simulink model "section_6_2_second_group"  (R2020a)
settings: Solver=ode45  StartTime=0.0  StopTime=50  RelTol=1e-5  EnableMultiTasking=on
(part 2 of 4)

== matlab function section_6_2_second_group/FUZZY3/fuzzy_logic_system1 ==
  data: aF output; x1 input; x2 input; x3 input; w input
function aF    = fcn(x1,x2,x3,w)
%%x1 5条模糊规则
delta=0.01;
ux1=zeros(5,1);
ux2=zeros(5,1);
ux3=zeros(5,1);
%%x1 5条模糊规则

h1=1;%%规则间距
if x1<=-2-delta
    ux1(1,1)=1;
end

if x1>=-2-delta&&x1<=-1-delta
    ux1(1,1)=0.5*sin(pi*(x1-(-2-delta))/h1+0.5*pi)+0.5;
end

if x1>=-2-delta&&x1<=0-delta
    ux1(2,1)=0.5*sin(pi*(x1-(-1-delta))/h1+0.5*pi)+0.5;
end

if x1>=-1-delta&&x1<=1-delta
    ux1(3,1)=0.5*sin(pi*(x1-(0-delta))/h1+0.5*pi)+0.5;
end

if x1>=0-delta&&x1<=2-delta
    ux1(4,1)=0.5*sin(pi*(x1-(1-delta))/h1+0.5*pi)+0.5;
end

if x1>=1-delta&&x1<=2-delta
    ux1(5,1)=0.5*sin(pi*(x1-(2-delta))/h1+0.5*pi)+0.5;
end

if x1>2-delta
    ux1(5,1)=1;
end


h2=1;%%规则间距
if x2<=-2-delta
    ux2(1,1)=1;
end

if x2>=-2-delta&&x2<=-1-delta
    ux2(1,1)=0.5*sin(pi*(x2-(-2-delta))/h2+0.5*pi)+0.5;
end

if x2>=-2-delta&&x2<=0-delta
    ux2(2,1)=0.5*sin(pi*(x2-(-1-delta))/h2+0.5*pi)+0.5;
end

if x2>=-1-delta&&x2<=1-delta
    ux2(3,1)=0.5*sin(pi*(x2-(0-delta))/h2+0.5*pi)+0.5;
end

if x2>=0-delta&&x2<=2-delta
    ux2(4,1)=0.5*sin(pi*(x2-(1-delta))/h2+0.5*pi)+0.5;
end

if x2>=1-delta&&x2<=2-delta
    ux2(5,1)=0.5*sin(pi*(x2-(2-delta))/h2+0.5*pi)+0.5;
end

if x2>2-delta
    ux2(5,1)=1;
end

h3=1;%%规则间距
if x3<=-2-delta
    ux3(1,1)=1;
end

if x3>=-2-delta&&x3<=-1-delta
    ux3(1,1)=0.5*sin(pi*(x3-(-2-delta))/h3+0.5*pi)+0.5;
end

if x3>=-2-delta&&x3<=0-delta
    ux3(2,1)=0.5*sin(pi*(x3-(-1-delta))/h3+0.5*pi)+0.5;
end

if x3>=-1-delta&&x3<=1-delta
    ux3(3,1)=0.5*sin(pi*(x3-(0-delta))/h3+0.5*pi)+0.5;
end

if x3>=0-delta&&x3<=2-delta
    ux3(4,1)=0.5*sin(pi*(x3-(1-delta))/h3+0.5*pi)+0.5;
end

if x3>=1-delta&&x3<=2-delta
    ux3(5,1)=0.5*sin(pi*(x3-(2-delta))/h3+0.5*pi)+0.5;
end

if x3>2-delta
    ux3(5,1)=1;
end



%中心平均解模糊
Basic=0;
for i1=1:5
    for i2=1:5
        for i3=1:5
            Basic=Basic+ux1(i1,1)*ux2(i2,1)*ux3(i3,1);
        end
    end
end

beta=zeros(5,5,5);
for i1=1:5
    for i2=1:5
        for i3=1:5
            beta(i1,i2,i3)=ux1(i1,1)*ux2(i2,1)*ux3(i3,1)/Basic;
        end
    end
end


aF=0;
for i1=1:5
    for i2=1:5
        for i3=1:5
            aF=aF+w(i1,i2,i3)*beta(i1,i2,i3); 
        end
    end
end

end

== matlab function section_6_2_second_group/FUZZY3/fuzzy_logic_system10 ==
  data: aF output; x1 input; x2 input; x3 input; w input
function aF    = fcn(x1,x2,x3,w)
%%x1 5条模糊规则
delta=0.01;
ux1=zeros(5,1);
ux2=zeros(5,1);
ux3=zeros(5,1);
%%x1 5条模糊规则

h1=1;%%规则间距
if x1<=-2-delta
    ux1(1,1)=1;
end

if x1>=-2-delta&&x1<=-1-delta
    ux1(1,1)=0.5*sin(pi*(x1-(-2-delta))/h1+0.5*pi)+0.5;
end

if x1>=-2-delta&&x1<=0-delta
    ux1(2,1)=0.5*sin(pi*(x1-(-1-delta))/h1+0.5*pi)+0.5;
end

if x1>=-1-delta&&x1<=1-delta
    ux1(3,1)=0.5*sin(pi*(x1-(0-delta))/h1+0.5*pi)+0.5;
end

if x1>=0-delta&&x1<=2-delta
    ux1(4,1)=0.5*sin(pi*(x1-(1-delta))/h1+0.5*pi)+0.5;
end

if x1>=1-delta&&x1<=2-delta
    ux1(5,1)=0.5*sin(pi*(x1-(2-delta))/h1+0.5*pi)+0.5;
end

if x1>2-delta
    ux1(5,1)=1;
end


h2=1;%%规则间距
if x2<=-2-delta
    ux2(1,1)=1;
end

if x2>=-2-delta&&x2<=-1-delta
    ux2(1,1)=0.5*sin(pi*(x2-(-2-delta))/h2+0.5*pi)+0.5;
end

if x2>=-2-delta&&x2<=0-delta
    ux2(2,1)=0.5*sin(pi*(x2-(-1-delta))/h2+0.5*pi)+0.5;
end

if x2>=-1-delta&&x2<=1-delta
    ux2(3,1)=0.5*sin(pi*(x2-(0-delta))/h2+0.5*pi)+0.5;
end

if x2>=0-delta&&x2<=2-delta
    ux2(4,1)=0.5*sin(pi*(x2-(1-delta))/h2+0.5*pi)+0.5;
end

if x2>=1-delta&&x2<=2-delta
    ux2(5,1)=0.5*sin(pi*(x2-(2-delta))/h2+0.5*pi)+0.5;
end

if x2>2-delta
    ux2(5,1)=1;
end

h3=1;%%规则间距
if x3<=-2-delta
    ux3(1,1)=1;
end

if x3>=-2-delta&&x3<=-1-delta
    ux3(1,1)=0.5*sin(pi*(x3-(-2-delta))/h3+0.5*pi)+0.5;
end

if x3>=-2-delta&&x3<=0-delta
    ux3(2,1)=0.5*sin(pi*(x3-(-1-delta))/h3+0.5*pi)+0.5;
end

if x3>=-1-delta&&x3<=1-delta
    ux3(3,1)=0.5*sin(pi*(x3-(0-delta))/h3+0.5*pi)+0.5;
end

if x3>=0-delta&&x3<=2-delta
    ux3(4,1)=0.5*sin(pi*(x3-(1-delta))/h3+0.5*pi)+0.5;
end

if x3>=1-delta&&x3<=2-delta
    ux3(5,1)=0.5*sin(pi*(x3-(2-delta))/h3+0.5*pi)+0.5;
end

if x3>2-delta
    ux3(5,1)=1;
end



%中心平均解模糊
Basic=0;
for i1=1:5
    for i2=1:5
        for i3=1:5
            Basic=Basic+ux1(i1,1)*ux2(i2,1)*ux3(i3,1);
        end
    end
end

beta=zeros(5,5,5);
for i1=1:5
    for i2=1:5
        for i3=1:5
            beta(i1,i2,i3)=ux1(i1,1)*ux2(i2,1)*ux3(i3,1)/Basic;
        end
    end
end


aF=0;
for i1=1:5
    for i2=1:5
        for i3=1:5
            aF=aF+w(i1,i2,i3)*beta(i1,i2,i3); 
        end
    end
end

end

== matlab function section_6_2_second_group/FUZZY3/fuzzy_logic_system2 ==
  data: aF output; x1 input; x2 input; x3 input; w input
function aF    = fcn(x1,x2,x3,w)
%%x1 5条模糊规则
delta=0.01;
ux1=zeros(5,1);
ux2=zeros(5,1);
ux3=zeros(5,1);
%%x1 5条模糊规则

h1=1;%%规则间距
if x1<=-2-delta
    ux1(1,1)=1;
end

if x1>=-2-delta&&x1<=-1-delta
    ux1(1,1)=0.5*sin(pi*(x1-(-2-delta))/h1+0.5*pi)+0.5;
end

if x1>=-2-delta&&x1<=0-delta
    ux1(2,1)=0.5*sin(pi*(x1-(-1-delta))/h1+0.5*pi)+0.5;
end

if x1>=-1-delta&&x1<=1-delta
    ux1(3,1)=0.5*sin(pi*(x1-(0-delta))/h1+0.5*pi)+0.5;
end

if x1>=0-delta&&x1<=2-delta
    ux1(4,1)=0.5*sin(pi*(x1-(1-delta))/h1+0.5*pi)+0.5;
end

if x1>=1-delta&&x1<=2-delta
    ux1(5,1)=0.5*sin(pi*(x1-(2-delta))/h1+0.5*pi)+0.5;
end

if x1>2-delta
    ux1(5,1)=1;
end


h2=1;%%规则间距
if x2<=-2-delta
    ux2(1,1)=1;
end

if x2>=-2-delta&&x2<=-1-delta
    ux2(1,1)=0.5*sin(pi*(x2-(-2-delta))/h2+0.5*pi)+0.5;
end

if x2>=-2-delta&&x2<=0-delta
    ux2(2,1)=0.5*sin(pi*(x2-(-1-delta))/h2+0.5*pi)+0.5;
end

if x2>=-1-delta&&x2<=1-delta
    ux2(3,1)=0.5*sin(pi*(x2-(0-delta))/h2+0.5*pi)+0.5;
end

if x2>=0-delta&&x2<=2-delta
    ux2(4,1)=0.5*sin(pi*(x2-(1-delta))/h2+0.5*pi)+0.5;
end

if x2>=1-delta&&x2<=2-delta
    ux2(5,1)=0.5*sin(pi*(x2-(2-delta))/h2+0.5*pi)+0.5;
end

if x2>2-delta
    ux2(5,1)=1;
end

h3=1;%%规则间距
if x3<=-2-delta
    ux3(1,1)=1;
end

if x3>=-2-delta&&x3<=-1-delta
    ux3(1,1)=0.5*sin(pi*(x3-(-2-delta))/h3+0.5*pi)+0.5;
end

if x3>=-2-delta&&x3<=0-delta
    ux3(2,1)=0.5*sin(pi*(x3-(-1-delta))/h3+0.5*pi)+0.5;
end

if x3>=-1-delta&&x3<=1-delta
    ux3(3,1)=0.5*sin(pi*(x3-(0-delta))/h3+0.5*pi)+0.5;
end

if x3>=0-delta&&x3<=2-delta
    ux3(4,1)=0.5*sin(pi*(x3-(1-delta))/h3+0.5*pi)+0.5;
end

if x3>=1-delta&&x3<=2-delta
    ux3(5,1)=0.5*sin(pi*(x3-(2-delta))/h3+0.5*pi)+0.5;
end

if x3>2-delta
    ux3(5,1)=1;
end



%中心平均解模糊
Basic=0;
for i1=1:5
    for i2=1:5
        for i3=1:5
            Basic=Basic+ux1(i1,1)*ux2(i2,1)*ux3(i3,1);
        end
    end
end

beta=zeros(5,5,5);
for i1=1:5
    for i2=1:5
        for i3=1:5
            beta(i1,i2,i3)=ux1(i1,1)*ux2(i2,1)*ux3(i3,1)/Basic;
        end
    end
end


aF=0;
for i1=1:5
    for i2=1:5
        for i3=1:5
            aF=aF+w(i1,i2,i3)*beta(i1,i2,i3); 
        end
    end
end

end

== matlab function section_6_2_second_group/FUZZY3/fuzzy_logic_system3 ==
  data: aF output; x1 input; x2 input; x3 input; w input
function aF    = fcn(x1,x2,x3,w)
%%x1 5条模糊规则
delta=0.01;
ux1=zeros(5,1);
ux2=zeros(5,1);
ux3=zeros(5,1);
%%x1 5条模糊规则

h1=1;%%规则间距
if x1<=-2-delta
    ux1(1,1)=1;
end

if x1>=-2-delta&&x1<=-1-delta
    ux1(1,1)=0.5*sin(pi*(x1-(-2-delta))/h1+0.5*pi)+0.5;
end

if x1>=-2-delta&&x1<=0-delta
    ux1(2,1)=0.5*sin(pi*(x1-(-1-delta))/h1+0.5*pi)+0.5;
end

if x1>=-1-delta&&x1<=1-delta
    ux1(3,1)=0.5*sin(pi*(x1-(0-delta))/h1+0.5*pi)+0.5;
end

if x1>=0-delta&&x1<=2-delta
    ux1(4,1)=0.5*sin(pi*(x1-(1-delta))/h1+0.5*pi)+0.5;
end

if x1>=1-delta&&x1<=2-delta
    ux1(5,1)=0.5*sin(pi*(x1-(2-delta))/h1+0.5*pi)+0.5;
end

if x1>2-delta
    ux1(5,1)=1;
end


h2=1;%%规则间距
if x2<=-2-delta
    ux2(1,1)=1;
end

if x2>=-2-delta&&x2<=-1-delta
    ux2(1,1)=0.5*sin(pi*(x2-(-2-delta))/h2+0.5*pi)+0.5;
end

if x2>=-2-delta&&x2<=0-delta
    ux2(2,1)=0.5*sin(pi*(x2-(-1-delta))/h2+0.5*pi)+0.5;
end

if x2>=-1-delta&&x2<=1-delta
    ux2(3,1)=0.5*sin(pi*(x2-(0-delta))/h2+0.5*pi)+0.5;
end

if x2>=0-delta&&x2<=2-delta
    ux2(4,1)=0.5*sin(pi*(x2-(1-delta))/h2+0.5*pi)+0.5;
end

if x2>=1-delta&&x2<=2-delta
    ux2(5,1)=0.5*sin(pi*(x2-(2-delta))/h2+0.5*pi)+0.5;
end

if x2>2-delta
    ux2(5,1)=1;
end

h3=1;%%规则间距
if x3<=-2-delta
    ux3(1,1)=1;
end

if x3>=-2-delta&&x3<=-1-delta
    ux3(1,1)=0.5*sin(pi*(x3-(-2-delta))/h3+0.5*pi)+0.5;
end

if x3>=-2-delta&&x3<=0-delta
    ux3(2,1)=0.5*sin(pi*(x3-(-1-delta))/h3+0.5*pi)+0.5;
end

if x3>=-1-delta&&x3<=1-delta
    ux3(3,1)=0.5*sin(pi*(x3-(0-delta))/h3+0.5*pi)+0.5;
end

if x3>=0-delta&&x3<=2-delta
    ux3(4,1)=0.5*sin(pi*(x3-(1-delta))/h3+0.5*pi)+0.5;
end

if x3>=1-delta&&x3<=2-delta
    ux3(5,1)=0.5*sin(pi*(x3-(2-delta))/h3+0.5*pi)+0.5;
end

if x3>2-delta
    ux3(5,1)=1;
end



%中心平均解模糊
Basic=0;
for i1=1:5
    for i2=1:5
        for i3=1:5
            Basic=Basic+ux1(i1,1)*ux2(i2,1)*ux3(i3,1);
        end
    end
end

beta=zeros(5,5,5);
for i1=1:5
    for i2=1:5
        for i3=1:5
            beta(i1,i2,i3)=ux1(i1,1)*ux2(i2,1)*ux3(i3,1)/Basic;
        end
    end
end


aF=0;
for i1=1:5
    for i2=1:5
        for i3=1:5
            aF=aF+w(i1,i2,i3)*beta(i1,i2,i3); 
        end
    end
end

end

== matlab function section_6_2_second_group/FUZZY3/fuzzy_logic_system4 ==
  data: aF output; x1 input; x2 input; x3 input; w input
function aF    = fcn(x1,x2,x3,w)
%%x1 5条模糊规则
delta=0.01;
ux1=zeros(5,1);
ux2=zeros(5,1);
ux3=zeros(5,1);
%%x1 5条模糊规则

h1=1;%%规则间距
if x1<=-2-delta
    ux1(1,1)=1;
end

if x1>=-2-delta&&x1<=-1-delta
    ux1(1,1)=0.5*sin(pi*(x1-(-2-delta))/h1+0.5*pi)+0.5;
end

if x1>=-2-delta&&x1<=0-delta
    ux1(2,1)=0.5*sin(pi*(x1-(-1-delta))/h1+0.5*pi)+0.5;
end

if x1>=-1-delta&&x1<=1-delta
    ux1(3,1)=0.5*sin(pi*(x1-(0-delta))/h1+0.5*pi)+0.5;
end

if x1>=0-delta&&x1<=2-delta
    ux1(4,1)=0.5*sin(pi*(x1-(1-delta))/h1+0.5*pi)+0.5;
end

if x1>=1-delta&&x1<=2-delta
    ux1(5,1)=0.5*sin(pi*(x1-(2-delta))/h1+0.5*pi)+0.5;
end

if x1>2-delta
    ux1(5,1)=1;
end


h2=1;%%规则间距
if x2<=-2-delta
    ux2(1,1)=1;
end

if x2>=-2-delta&&x2<=-1-delta
    ux2(1,1)=0.5*sin(pi*(x2-(-2-delta))/h2+0.5*pi)+0.5;
end

if x2>=-2-delta&&x2<=0-delta
    ux2(2,1)=0.5*sin(pi*(x2-(-1-delta))/h2+0.5*pi)+0.5;
end

if x2>=-1-delta&&x2<=1-delta
    ux2(3,1)=0.5*sin(pi*(x2-(0-delta))/h2+0.5*pi)+0.5;
end

if x2>=0-delta&&x2<=2-delta
    ux2(4,1)=0.5*sin(pi*(x2-(1-delta))/h2+0.5*pi)+0.5;
end

if x2>=1-delta&&x2<=2-delta
    ux2(5,1)=0.5*sin(pi*(x2-(2-delta))/h2+0.5*pi)+0.5;
end

if x2>2-delta
    ux2(5,1)=1;
end

h3=1;%%规则间距
if x3<=-2-delta
    ux3(1,1)=1;
end

if x3>=-2-delta&&x3<=-1-delta
    ux3(1,1)=0.5*sin(pi*(x3-(-2-delta))/h3+0.5*pi)+0.5;
end

if x3>=-2-delta&&x3<=0-delta
    ux3(2,1)=0.5*sin(pi*(x3-(-1-delta))/h3+0.5*pi)+0.5;
end

if x3>=-1-delta&&x3<=1-delta
    ux3(3,1)=0.5*sin(pi*(x3-(0-delta))/h3+0.5*pi)+0.5;
end

if x3>=0-delta&&x3<=2-delta
    ux3(4,1)=0.5*sin(pi*(x3-(1-delta))/h3+0.5*pi)+0.5;
end

if x3>=1-delta&&x3<=2-delta
    ux3(5,1)=0.5*sin(pi*(x3-(2-delta))/h3+0.5*pi)+0.5;
end

if x3>2-delta
    ux3(5,1)=1;
end



%中心平均解模糊
Basic=0;
for i1=1:5
    for i2=1:5
        for i3=1:5
            Basic=Basic+ux1(i1,1)*ux2(i2,1)*ux3(i3,1);
        end
    end
end

beta=zeros(5,5,5);
for i1=1:5
    for i2=1:5
        for i3=1:5
            beta(i1,i2,i3)=ux1(i1,1)*ux2(i2,1)*ux3(i3,1)/Basic;
        end
    end
end


aF=0;
for i1=1:5
    for i2=1:5
        for i3=1:5
            aF=aF+w(i1,i2,i3)*beta(i1,i2,i3); 
        end
    end
end

end

== matlab function section_6_2_second_group/FUZZY3/fuzzy_logic_system5 ==
  data: aF output; x1 input; x2 input; x3 input; w input
function aF    = fcn(x1,x2,x3,w)
%%x1 5条模糊规则
delta=0.01;
ux1=zeros(5,1);
ux2=zeros(5,1);
ux3=zeros(5,1);
%%x1 5条模糊规则

h1=1;%%规则间距
if x1<=-2-delta
    ux1(1,1)=1;
end

if x1>=-2-delta&&x1<=-1-delta
    ux1(1,1)=0.5*sin(pi*(x1-(-2-delta))/h1+0.5*pi)+0.5;
end

if x1>=-2-delta&&x1<=0-delta
    ux1(2,1)=0.5*sin(pi*(x1-(-1-delta))/h1+0.5*pi)+0.5;
end

if x1>=-1-delta&&x1<=1-delta
    ux1(3,1)=0.5*sin(pi*(x1-(0-delta))/h1+0.5*pi)+0.5;
end

if x1>=0-delta&&x1<=2-delta
    ux1(4,1)=0.5*sin(pi*(x1-(1-delta))/h1+0.5*pi)+0.5;
end

if x1>=1-delta&&x1<=2-delta
    ux1(5,1)=0.5*sin(pi*(x1-(2-delta))/h1+0.5*pi)+0.5;
end

if x1>2-delta
    ux1(5,1)=1;
end


h2=1;%%规则间距
if x2<=-2-delta
    ux2(1,1)=1;
end

if x2>=-2-delta&&x2<=-1-delta
    ux2(1,1)=0.5*sin(pi*(x2-(-2-delta))/h2+0.5*pi)+0.5;
end

if x2>=-2-delta&&x2<=0-delta
    ux2(2,1)=0.5*sin(pi*(x2-(-1-delta))/h2+0.5*pi)+0.5;
end

if x2>=-1-delta&&x2<=1-delta
    ux2(3,1)=0.5*sin(pi*(x2-(0-delta))/h2+0.5*pi)+0.5;
end

if x2>=0-delta&&x2<=2-delta
    ux2(4,1)=0.5*sin(pi*(x2-(1-delta))/h2+0.5*pi)+0.5;
end

if x2>=1-delta&&x2<=2-delta
    ux2(5,1)=0.5*sin(pi*(x2-(2-delta))/h2+0.5*pi)+0.5;
end

if x2>2-delta
    ux2(5,1)=1;
end

h3=1;%%规则间距
if x3<=-2-delta
    ux3(1,1)=1;
end

if x3>=-2-delta&&x3<=-1-delta
    ux3(1,1)=0.5*sin(pi*(x3-(-2-delta))/h3+0.5*pi)+0.5;
end

if x3>=-2-delta&&x3<=0-delta
    ux3(2,1)=0.5*sin(pi*(x3-(-1-delta))/h3+0.5*pi)+0.5;
end

if x3>=-1-delta&&x3<=1-delta
    ux3(3,1)=0.5*sin(pi*(x3-(0-delta))/h3+0.5*pi)+0.5;
end

if x3>=0-delta&&x3<=2-delta
    ux3(4,1)=0.5*sin(pi*(x3-(1-delta))/h3+0.5*pi)+0.5;
end

if x3>=1-delta&&x3<=2-delta
    ux3(5,1)=0.5*sin(pi*(x3-(2-delta))/h3+0.5*pi)+0.5;
end

if x3>2-delta
    ux3(5,1)=1;
end



%中心平均解模糊
Basic=0;
for i1=1:5
    for i2=1:5
        for i3=1:5
            Basic=Basic+ux1(i1,1)*ux2(i2,1)*ux3(i3,1);
        end
    end
end

beta=zeros(5,5,5);
for i1=1:5
    for i2=1:5
        for i3=1:5
            beta(i1,i2,i3)=ux1(i1,1)*ux2(i2,1)*ux3(i3,1)/Basic;
        end
    end
end


aF=0;
for i1=1:5
    for i2=1:5
        for i3=1:5
            aF=aF+w(i1,i2,i3)*beta(i1,i2,i3); 
        end
    end
end

end

== matlab function section_6_2_second_group/FUZZY3/fuzzy_logic_system6 ==
  data: aF output; x1 input; x2 input; x3 input; w input
function aF    = fcn(x1,x2,x3,w)
%%x1 5条模糊规则
delta=0.01;
ux1=zeros(5,1);
ux2=zeros(5,1);
ux3=zeros(5,1);
%%x1 5条模糊规则

h1=1;%%规则间距
if x1<=-2-delta
    ux1(1,1)=1;
end

if x1>=-2-delta&&x1<=-1-delta
    ux1(1,1)=0.5*sin(pi*(x1-(-2-delta))/h1+0.5*pi)+0.5;
end

if x1>=-2-delta&&x1<=0-delta
    ux1(2,1)=0.5*sin(pi*(x1-(-1-delta))/h1+0.5*pi)+0.5;
end

if x1>=-1-delta&&x1<=1-delta
    ux1(3,1)=0.5*sin(pi*(x1-(0-delta))/h1+0.5*pi)+0.5;
end

if x1>=0-delta&&x1<=2-delta
    ux1(4,1)=0.5*sin(pi*(x1-(1-delta))/h1+0.5*pi)+0.5;
end

if x1>=1-delta&&x1<=2-delta
    ux1(5,1)=0.5*sin(pi*(x1-(2-delta))/h1+0.5*pi)+0.5;
end

if x1>2-delta
    ux1(5,1)=1;
end


h2=1;%%规则间距
if x2<=-2-delta
    ux2(1,1)=1;
end

if x2>=-2-delta&&x2<=-1-delta
    ux2(1,1)=0.5*sin(pi*(x2-(-2-delta))/h2+0.5*pi)+0.5;
end

if x2>=-2-delta&&x2<=0-delta
    ux2(2,1)=0.5*sin(pi*(x2-(-1-delta))/h2+0.5*pi)+0.5;
end

if x2>=-1-delta&&x2<=1-delta
    ux2(3,1)=0.5*sin(pi*(x2-(0-delta))/h2+0.5*pi)+0.5;
end

if x2>=0-delta&&x2<=2-delta
    ux2(4,1)=0.5*sin(pi*(x2-(1-delta))/h2+0.5*pi)+0.5;
end

if x2>=1-delta&&x2<=2-delta
    ux2(5,1)=0.5*sin(pi*(x2-(2-delta))/h2+0.5*pi)+0.5;
end

if x2>2-delta
    ux2(5,1)=1;
end

h3=1;%%规则间距
if x3<=-2-delta
    ux3(1,1)=1;
end

if x3>=-2-delta&&x3<=-1-delta
    ux3(1,1)=0.5*sin(pi*(x3-(-2-delta))/h3+0.5*pi)+0.5;
end

if x3>=-2-delta&&x3<=0-delta
    ux3(2,1)=0.5*sin(pi*(x3-(-1-delta))/h3+0.5*pi)+0.5;
end

if x3>=-1-delta&&x3<=1-delta
    ux3(3,1)=0.5*sin(pi*(x3-(0-delta))/h3+0.5*pi)+0.5;
end

if x3>=0-delta&&x3<=2-delta
    ux3(4,1)=0.5*sin(pi*(x3-(1-delta))/h3+0.5*pi)+0.5;
end

if x3>=1-delta&&x3<=2-delta
    ux3(5,1)=0.5*sin(pi*(x3-(2-delta))/h3+0.5*pi)+0.5;
end

if x3>2-delta
    ux3(5,1)=1;
end



%中心平均解模糊
Basic=0;
for i1=1:5
    for i2=1:5
        for i3=1:5
            Basic=Basic+ux1(i1,1)*ux2(i2,1)*ux3(i3,1);
        end
    end
end

beta=zeros(5,5,5);
for i1=1:5
    for i2=1:5
        for i3=1:5
            beta(i1,i2,i3)=ux1(i1,1)*ux2(i2,1)*ux3(i3,1)/Basic;
        end
    end
end


aF=0;
for i1=1:5
    for i2=1:5
        for i3=1:5
            aF=aF+w(i1,i2,i3)*beta(i1,i2,i3); 
        end
    end
end

end

== matlab function section_6_2_second_group/FUZZY3/fuzzy_logic_system7 ==
  data: aF output; x1 input; x2 input; x3 input; w input
function aF    = fcn(x1,x2,x3,w)
%%x1 5条模糊规则
delta=0.01;
ux1=zeros(5,1);
ux2=zeros(5,1);
ux3=zeros(5,1);
%%x1 5条模糊规则

h1=1;%%规则间距
if x1<=-2-delta
    ux1(1,1)=1;
end

if x1>=-2-delta&&x1<=-1-delta
    ux1(1,1)=0.5*sin(pi*(x1-(-2-delta))/h1+0.5*pi)+0.5;
end

if x1>=-2-delta&&x1<=0-delta
    ux1(2,1)=0.5*sin(pi*(x1-(-1-delta))/h1+0.5*pi)+0.5;
end

if x1>=-1-delta&&x1<=1-delta
    ux1(3,1)=0.5*sin(pi*(x1-(0-delta))/h1+0.5*pi)+0.5;
end

if x1>=0-delta&&x1<=2-delta
    ux1(4,1)=0.5*sin(pi*(x1-(1-delta))/h1+0.5*pi)+0.5;
end

if x1>=1-delta&&x1<=2-delta
    ux1(5,1)=0.5*sin(pi*(x1-(2-delta))/h1+0.5*pi)+0.5;
end

if x1>2-delta
    ux1(5,1)=1;
end


h2=1;%%规则间距
if x2<=-2-delta
    ux2(1,1)=1;
end

if x2>=-2-delta&&x2<=-1-delta
    ux2(1,1)=0.5*sin(pi*(x2-(-2-delta))/h2+0.5*pi)+0.5;
end

if x2>=-2-delta&&x2<=0-delta
    ux2(2,1)=0.5*sin(pi*(x2-(-1-delta))/h2+0.5*pi)+0.5;
end

if x2>=-1-delta&&x2<=1-delta
    ux2(3,1)=0.5*sin(pi*(x2-(0-delta))/h2+0.5*pi)+0.5;
end

if x2>=0-delta&&x2<=2-delta
    ux2(4,1)=0.5*sin(pi*(x2-(1-delta))/h2+0.5*pi)+0.5;
end

if x2>=1-delta&&x2<=2-delta
    ux2(5,1)=0.5*sin(pi*(x2-(2-delta))/h2+0.5*pi)+0.5;
end

if x2>2-delta
    ux2(5,1)=1;
end

h3=1;%%规则间距
if x3<=-2-delta
    ux3(1,1)=1;
end

if x3>=-2-delta&&x3<=-1-delta
    ux3(1,1)=0.5*sin(pi*(x3-(-2-delta))/h3+0.5*pi)+0.5;
end

if x3>=-2-delta&&x3<=0-delta
    ux3(2,1)=0.5*sin(pi*(x3-(-1-delta))/h3+0.5*pi)+0.5;
end

if x3>=-1-delta&&x3<=1-delta
    ux3(3,1)=0.5*sin(pi*(x3-(0-delta))/h3+0.5*pi)+0.5;
end

if x3>=0-delta&&x3<=2-delta
    ux3(4,1)=0.5*sin(pi*(x3-(1-delta))/h3+0.5*pi)+0.5;
end

if x3>=1-delta&&x3<=2-delta
    ux3(5,1)=0.5*sin(pi*(x3-(2-delta))/h3+0.5*pi)+0.5;
end

if x3>2-delta
    ux3(5,1)=1;
end



%中心平均解模糊
Basic=0;
for i1=1:5
    for i2=1:5
        for i3=1:5
            Basic=Basic+ux1(i1,1)*ux2(i2,1)*ux3(i3,1);
        end
    end
end

beta=zeros(5,5,5);
for i1=1:5
    for i2=1:5
        for i3=1:5
            beta(i1,i2,i3)=ux1(i1,1)*ux2(i2,1)*ux3(i3,1)/Basic;
        end
    end
end


aF=0;
for i1=1:5
    for i2=1:5
        for i3=1:5
            aF=aF+w(i1,i2,i3)*beta(i1,i2,i3); 
        end
    end
end

end

== matlab function section_6_2_second_group/FUZZY3/fuzzy_logic_system8 ==
  data: aF output; x1 input; x2 input; x3 input; w input
function aF    = fcn(x1,x2,x3,w)
%%x1 5条模糊规则
delta=0.01;
ux1=zeros(5,1);
ux2=zeros(5,1);
ux3=zeros(5,1);
%%x1 5条模糊规则

h1=1;%%规则间距
if x1<=-2-delta
    ux1(1,1)=1;
end

if x1>=-2-delta&&x1<=-1-delta
    ux1(1,1)=0.5*sin(pi*(x1-(-2-delta))/h1+0.5*pi)+0.5;
end

if x1>=-2-delta&&x1<=0-delta
    ux1(2,1)=0.5*sin(pi*(x1-(-1-delta))/h1+0.5*pi)+0.5;
end

if x1>=-1-delta&&x1<=1-delta
    ux1(3,1)=0.5*sin(pi*(x1-(0-delta))/h1+0.5*pi)+0.5;
end

if x1>=0-delta&&x1<=2-delta
    ux1(4,1)=0.5*sin(pi*(x1-(1-delta))/h1+0.5*pi)+0.5;
end

if x1>=1-delta&&x1<=2-delta
    ux1(5,1)=0.5*sin(pi*(x1-(2-delta))/h1+0.5*pi)+0.5;
end

if x1>2-delta
    ux1(5,1)=1;
end


h2=1;%%规则间距
if x2<=-2-delta
    ux2(1,1)=1;
end

if x2>=-2-delta&&x2<=-1-delta
    ux2(1,1)=0.5*sin(pi*(x2-(-2-delta))/h2+0.5*pi)+0.5;
end

if x2>=-2-delta&&x2<=0-delta
    ux2(2,1)=0.5*sin(pi*(x2-(-1-delta))/h2+0.5*pi)+0.5;
end

if x2>=-1-delta&&x2<=1-delta
    ux2(3,1)=0.5*sin(pi*(x2-(0-delta))/h2+0.5*pi)+0.5;
end

if x2>=0-delta&&x2<=2-delta
    ux2(4,1)=0.5*sin(pi*(x2-(1-delta))/h2+0.5*pi)+0.5;
end

if x2>=1-delta&&x2<=2-delta
    ux2(5,1)=0.5*sin(pi*(x2-(2-delta))/h2+0.5*pi)+0.5;
end

if x2>2-delta
    ux2(5,1)=1;
end

h3=1;%%规则间距
if x3<=-2-delta
    ux3(1,1)=1;
end

if x3>=-2-delta&&x3<=-1-delta
    ux3(1,1)=0.5*sin(pi*(x3-(-2-delta))/h3+0.5*pi)+0.5;
end

if x3>=-2-delta&&x3<=0-delta
    ux3(2,1)=0.5*sin(pi*(x3-(-1-delta))/h3+0.5*pi)+0.5;
end

if x3>=-1-delta&&x3<=1-delta
    ux3(3,1)=0.5*sin(pi*(x3-(0-delta))/h3+0.5*pi)+0.5;
end

if x3>=0-delta&&x3<=2-delta
    ux3(4,1)=0.5*sin(pi*(x3-(1-delta))/h3+0.5*pi)+0.5;
end

if x3>=1-delta&&x3<=2-delta
    ux3(5,1)=0.5*sin(pi*(x3-(2-delta))/h3+0.5*pi)+0.5;
end

if x3>2-delta
    ux3(5,1)=1;
end



%中心平均解模糊
Basic=0;
for i1=1:5
    for i2=1:5
        for i3=1:5
            Basic=Basic+ux1(i1,1)*ux2(i2,1)*ux3(i3,1);
        end
    end
end

beta=zeros(5,5,5);
for i1=1:5
    for i2=1:5
        for i3=1:5
            beta(i1,i2,i3)=ux1(i1,1)*ux2(i2,1)*ux3(i3,1)/Basic;
        end
    end
end


aF=0;
for i1=1:5
    for i2=1:5
        for i3=1:5
            aF=aF+w(i1,i2,i3)*beta(i1,i2,i3); 
        end
    end
end

end

== matlab function section_6_2_second_group/delta1_adaptive ==
  data: w input; z11 input; Kv_dot output
function Kv_dot  = fcn(w,z11)
Kv_dot=w*abs(z11)^2;
end

== matlab function section_6_2_second_group/delta2_adaptive ==
  data: w input; z21 input; Kv_dot output
function Kv_dot  = fcn(w,z21)
Kv_dot=w*abs(z21)^2;
end

== matlab function section_6_2_second_group/delta3_adaptive ==
  data: w input; z31 input; Kv_dot output
function Kv_dot  = fcn(w,z31)
Kv_dot=w*abs(z31)^2;
end

== matlab function section_6_2_second_group/Kv12_adaptive1 ==
  data: w input; z13 input; Kv_dot output
function Kv_dot  = fcn(w,z13)
Kv_dot=w*abs(z13);
end

== matlab function section_6_2_second_group/Kv21_adaptive1 ==
  data: w input; z22 input; Kv_dot output
function Kv_dot  = fcn(w,z22)
Kv_dot=w*abs(z22);
end

== matlab function section_6_2_second_group/Kv22_adaptive2 ==
  data: w input; z23 input; Kv_dot output
function Kv_dot  = fcn(w,z23)
Kv_dot=w*abs(z23);
end

== matlab function section_6_2_second_group/Kv31_adaptive2 ==
  data: w input; z32 input; Kv_dot output
function Kv_dot  = fcn(w,z32)
Kv_dot=w*abs(z32);
end

== matlab function section_6_2_second_group/Kv32_adaptive3 ==
  data: w input; z33 input; Kv_dot output
function Kv_dot  = fcn(w,z33)
Kv_dot=w*abs(z33);
end

== matlab function section_6_2_second_group/Fuzzy_intial2 ==
  data: F11 output; x11 input; x12 input; x13 input; x21 input; x22 input; x23 input; x31 input; x32 input; x33 input; F12 output; F13 output; F21 output; F22 output; F23 output; F31 output; F32 output; F33 output
function [F11,F12,F13,F21,F22,F23,F31,F32,F33]    = fcn(x11,x12,x13,x21,x22,x23,x31,x32,x33)

F11=x11+1;
F12=x12+1;
F13=x13+1;
F21=x21+1;
F22=x22+1;
F23=x23+1;
F31=x31+1;
F32=x32+1;
F33=x33+1;

end

== matlab function section_6_2_second_group/Fuzzy_intial3 ==
  data: F11 output; x11 input; x12 input; x13 input; x21 input; x22 input; x23 input; x31 input; x32 input; x33 input; F12 output; F13 output; F21 output; F22 output; F23 output; F31 output; F32 output; F33 output
function [F11,F12,F13,F21,F22,F23,F31,F32,F33]    = fcn(x11,x12,x13,x21,x22,x23,x31,x32,x33)

F11=x11+1;
F12=x12+1;
F13=x13+1;
F21=x21+1;
F22=x22+1;
F23=x23+1;
F31=x31+1;
F32=x32+1;
F33=x33+1;


end

== matlab function section_6_2_second_group/FUZZY1/2D-3D2 ==
  data: y output; x input
function y  = fcn(x)
y=zeros(5,5,5);

for i=1:5
    for j=1:5
        for k=1:5
            y(i,j,k)=x(5*(k-1)+i,j);
        end
    end
end

end

== matlab function section_6_2_second_group/Kv11_adaptive1 ==
  data: dag input; dag_dot output; w input
function dag_dot  = fcn(dag,w)
dagd=0.1;
dag_dot=w*(dagd-dag);
end

== matlab function section_6_2_second_group/FUZZYB/2D-3D1 ==
  data: y output; x input
function y  = fcn(x)
y=zeros(5,5,5);

for i=1:5
    for j=1:5
        for k=1:5
            y(i,j,k)=x(5*(k-1)+i,j);
        end
    end
end

end

== matlab function section_6_2_second_group/Fuzzy_intial4 ==
  data: BF1 output; x1 input; x2 input; x3 input; BF2 output; BF3 output
function [BF1,BF2,BF3]    = fcn(x1,x2,x3)

BF1=x1+0.2;
BF2=x2+0.2;
BF3=x3+0.2;


end

== matlab function section_6_2_second_group/error ==
  data: xd input; e1 output; x1 input; x2 input; x3 input; e2 output; e3 output
function [e1,e2,e3]  = fcn(xd,x1,x2,x3)

e1=x1-xd;
e2=x2-xd;
e3=x3-xd;

end

== matlab function section_6_2_second_group/FUZZYB/2D-3D4 ==
  data: y output; x input
function y  = fcn(x)
y=zeros(5,5,5);

for i=1:5
    for j=1:5
        for k=1:5
            y(i,j,k)=x(5*(k-1)+i,j);
        end
    end
end

end

== matlab function section_6_2_second_group/FUZZYB/2D-3D7 ==
  data: y output; x input
function y  = fcn(x)
y=zeros(5,5,5);

for i=1:5
    for j=1:5
        for k=1:5
            y(i,j,k)=x(5*(k-1)+i,j);
        end
    end
end

end

== matlab function section_6_2_second_group/FUZZYB/3D-2D1 ==
  data: y output; x input
function y  = fcn(x)
y=zeros(25,5);

for i=1:5
    for j=1:5
        for k=1:5
            y(5*(k-1)+i,j)=x(i,j,k);
        end
    end
end


end

== matlab function section_6_2_second_group/FUZZYB/3D-2D4 ==
  data: y output; x input
function y  = fcn(x)
y=zeros(25,5);

for i=1:5
    for j=1:5
        for k=1:5
            y(5*(k-1)+i,j)=x(i,j,k);
        end
    end
end


end

== matlab function section_6_2_second_group/follower1 ==
  data: x1 input; x2 input; x3 input; x1dot output; u1 input; x2dot output; x3dot output
function [x1dot,x2dot,x3dot] = fcn(x1,x2,x3,u1)

f11=2*(exp(20*x2^2)-x2^2)/(exp(20*x2^2)+x2^2);
f12=6*tanh(x1+10*x3^2);
f13=170*tanh(x2+10*u1^2); 

g11=x3^2/(1+x1^2+x2^2)+sin(x3);
g12=-x2;
g13=x3^2/(1+x1^2+x2^2);

x1dot=f11*sin(x2+x3)+g11;
x2dot=f12*x3+g12;
x3dot=f13*sin(u1/15)+g13;

% x1dot=x1+x2+x3;
% x2dot=x1+x2+x3;
% x3dot=x1+x2+x3+u1;

end

== matlab function section_6_2_second_group/FUZZYB/3D-2D7 ==
  data: y output; x input
function y  = fcn(x)
y=zeros(25,5);

for i=1:5
    for j=1:5
        for k=1:5
            y(5*(k-1)+i,j)=x(i,j,k);
        end
    end
end


end

== matlab function section_6_2_second_group/FUZZYB/fuzzy_adaptive_law1 ==
  data: wdot output; x1 input; x2 input; x3 input; z3 input; w input; u1 input
function wdot   = fcn(x1,x2,x3,z3,w,u1)
delta=0.01;
ux1=zeros(5,1);
ux2=zeros(5,1);
ux3=zeros(5,1);
%%x1 5条模糊规则

z=zeros(5,6);
for j=1:5
    z(j,1)=-2+j-delta;
end
for j=6:10
    z(j-5,2)=-2+(j-5)-delta;
end
for j=11:15
    z(j-10,3)=-2+(j-10)-delta;
end

h1=1;%%规则间距
if x1<=-2-delta
    ux1(1,1)=1;
end

if x1>=-2-delta&&x1<=-1-delta
    ux1(1,1)=0.5*sin(pi*(x1-(-2-delta))/h1+0.5*pi)+0.5;
end

if x1>=-2-delta&&x1<=0-delta
    ux1(2,1)=0.5*sin(pi*(x1-(-1-delta))/h1+0.5*pi)+0.5;
end

if x1>=-1-delta&&x1<=1-delta
    ux1(3,1)=0.5*sin(pi*(x1-(0-delta))/h1+0.5*pi)+0.5;
end

if x1>=0-delta&&x1<=2-delta
    ux1(4,1)=0.5*sin(pi*(x1-(1-delta))/h1+0.5*pi)+0.5;
end

if x1>=1-delta&&x1<=2-delta
    ux1(5,1)=0.5*sin(pi*(x1-(2-delta))/h1+0.5*pi)+0.5;
end

if x1>2-delta
    ux1(5,1)=1;
end


h2=1;%%规则间距
if x2<=-2-delta
    ux2(1,1)=1;
end

if x2>=-2-delta&&x2<=-1-delta
    ux2(1,1)=0.5*sin(pi*(x2-(-2-delta))/h2+0.5*pi)+0.5;
end

if x2>=-2-delta&&x2<=0-delta
    ux2(2,1)=0.5*sin(pi*(x2-(-1-delta))/h2+0.5*pi)+0.5;
end

if x2>=-1-delta&&x2<=1-delta
    ux2(3,1)=0.5*sin(pi*(x2-(0-delta))/h2+0.5*pi)+0.5;
end

if x2>=0-delta&&x2<=2-delta
    ux2(4,1)=0.5*sin(pi*(x2-(1-delta))/h2+0.5*pi)+0.5;
end

if x2>=1-delta&&x2<=2-delta
    ux2(5,1)=0.5*sin(pi*(x2-(2-delta))/h2+0.5*pi)+0.5;
end

if x2>2-delta
    ux2(5,1)=1;
end

h3=1;%%规则间距
if x3<=-2-delta
    ux3(1,1)=1;
end

if x3>=-2-delta&&x3<=-1-delta
    ux3(1,1)=0.5*sin(pi*(x3-(-2-delta))/h3+0.5*pi)+0.5;
end

if x3>=-2-delta&&x3<=0-delta
    ux3(2,1)=0.5*sin(pi*(x3-(-1-delta))/h3+0.5*pi)+0.5;
end

if x3>=-1-delta&&x3<=1-delta
    ux3(3,1)=0.5*sin(pi*(x3-(0-delta))/h3+0.5*pi)+0.5;
end

if x3>=0-delta&&x3<=2-delta
    ux3(4,1)=0.5*sin(pi*(x3-(1-delta))/h3+0.5*pi)+0.5;
end

if x3>=1-delta&&x3<=2-delta
    ux3(5,1)=0.5*sin(pi*(x3-(2-delta))/h3+0.5*pi)+0.5;
end

if x3>2-delta
    ux3(5,1)=1;
end


%中心平均解模糊
Basic=0;
for i1=1:5
    for i2=1:5
        for i3=1:5
            Basic=Basic+ux1(i1,1)*ux2(i2,1)*ux3(i3,1);  
        end
    end
end

beta=zeros(5,5,5);
for i1=1:5
    for i2=1:5
        for i3=1:5
            beta(i1,i2,i3)=ux1(i1,1)*ux2(i2,1)*ux3(i3,1)/Basic;
        end
    end
end

wdot=zeros(5,5,5);
for i1=1:5
    for i2=1:5
        for i3=1:5
            wdot(i1,i2,i3)=w*beta(i1,i2,i3)*z3*u1;
        end
    end
end

end

== matlab function section_6_2_second_group/FUZZYB/fuzzy_adaptive_law2 ==
  data: wdot output; x1 input; x2 input; x3 input; z3 input; w input; u1 input
function wdot   = fcn(x1,x2,x3,z3,w,u1)
delta=0.01;
ux1=zeros(5,1);
ux2=zeros(5,1);
ux3=zeros(5,1);
%%x1 5条模糊规则

z=zeros(5,6);
for j=1:5
    z(j,1)=-2+j-delta;
end
for j=6:10
    z(j-5,2)=-2+(j-5)-delta;
end
for j=11:15
    z(j-10,3)=-2+(j-10)-delta;
end

h1=1;%%规则间距
if x1<=-2-delta
    ux1(1,1)=1;
end

if x1>=-2-delta&&x1<=-1-delta
    ux1(1,1)=0.5*sin(pi*(x1-(-2-delta))/h1+0.5*pi)+0.5;
end

if x1>=-2-delta&&x1<=0-delta
    ux1(2,1)=0.5*sin(pi*(x1-(-1-delta))/h1+0.5*pi)+0.5;
end

if x1>=-1-delta&&x1<=1-delta
    ux1(3,1)=0.5*sin(pi*(x1-(0-delta))/h1+0.5*pi)+0.5;
end

if x1>=0-delta&&x1<=2-delta
    ux1(4,1)=0.5*sin(pi*(x1-(1-delta))/h1+0.5*pi)+0.5;
end

if x1>=1-delta&&x1<=2-delta
    ux1(5,1)=0.5*sin(pi*(x1-(2-delta))/h1+0.5*pi)+0.5;
end

if x1>2-delta
    ux1(5,1)=1;
end


h2=1;%%规则间距
if x2<=-2-delta
    ux2(1,1)=1;
end

if x2>=-2-delta&&x2<=-1-delta
    ux2(1,1)=0.5*sin(pi*(x2-(-2-delta))/h2+0.5*pi)+0.5;
end

if x2>=-2-delta&&x2<=0-delta
    ux2(2,1)=0.5*sin(pi*(x2-(-1-delta))/h2+0.5*pi)+0.5;
end

if x2>=-1-delta&&x2<=1-delta
    ux2(3,1)=0.5*sin(pi*(x2-(0-delta))/h2+0.5*pi)+0.5;
end

if x2>=0-delta&&x2<=2-delta
    ux2(4,1)=0.5*sin(pi*(x2-(1-delta))/h2+0.5*pi)+0.5;
end

if x2>=1-delta&&x2<=2-delta
    ux2(5,1)=0.5*sin(pi*(x2-(2-delta))/h2+0.5*pi)+0.5;
end

if x2>2-delta
    ux2(5,1)=1;
end

h3=1;%%规则间距
if x3<=-2-delta
    ux3(1,1)=1;
end

if x3>=-2-delta&&x3<=-1-delta
    ux3(1,1)=0.5*sin(pi*(x3-(-2-delta))/h3+0.5*pi)+0.5;
end

if x3>=-2-delta&&x3<=0-delta
    ux3(2,1)=0.5*sin(pi*(x3-(-1-delta))/h3+0.5*pi)+0.5;
end

if x3>=-1-delta&&x3<=1-delta
    ux3(3,1)=0.5*sin(pi*(x3-(0-delta))/h3+0.5*pi)+0.5;
end

if x3>=0-delta&&x3<=2-delta
    ux3(4,1)=0.5*sin(pi*(x3-(1-delta))/h3+0.5*pi)+0.5;
end

if x3>=1-delta&&x3<=2-delta
    ux3(5,1)=0.5*sin(pi*(x3-(2-delta))/h3+0.5*pi)+0.5;
end

if x3>2-delta
    ux3(5,1)=1;
end


%中心平均解模糊
Basic=0;
for i1=1:5
    for i2=1:5
        for i3=1:5
            Basic=Basic+ux1(i1,1)*ux2(i2,1)*ux3(i3,1);  
        end
    end
end

beta=zeros(5,5,5);
for i1=1:5
    for i2=1:5
        for i3=1:5
            beta(i1,i2,i3)=ux1(i1,1)*ux2(i2,1)*ux3(i3,1)/Basic;
        end
    end
end

wdot=zeros(5,5,5);
for i1=1:5
    for i2=1:5
        for i3=1:5
            wdot(i1,i2,i3)=w*beta(i1,i2,i3)*z3*u1;
        end
    end
end

end

== matlab function section_6_2_second_group/Fuzzy_intial1 ==
  data: F11 output; x11 input; x12 input; x13 input; x21 input; x22 input; x23 input; x31 input; x32 input; x33 input; F12 output; F13 output; F21 output; F22 output; F23 output; F31 output; F32 output; F33 output
function [F11,F12,F13,F21,F22,F23,F31,F32,F33]    = fcn(x11,x12,x13,x21,x22,x23,x31,x32,x33)

F11=x11+1;
F12=x12+1;
F13=x13+1;
F21=x21+1;
F22=x22+1;
F23=x23+1;
F31=x31+1;
F32=x32+1;
F33=x33+1;

end

== matlab function section_6_2_second_group/FUZZYB/fuzzy_adaptive_law3 ==
  data: wdot output; x1 input; x2 input; x3 input; z3 input; w input; u1 input
function wdot   = fcn(x1,x2,x3,z3,w,u1)
delta=0.01;
ux1=zeros(5,1);
ux2=zeros(5,1);
ux3=zeros(5,1);
%%x1 5条模糊规则

z=zeros(5,6);
for j=1:5
    z(j,1)=-2+j-delta;
end
for j=6:10
    z(j-5,2)=-2+(j-5)-delta;
end
for j=11:15
    z(j-10,3)=-2+(j-10)-delta;
end

h1=1;%%规则间距
if x1<=-2-delta
    ux1(1,1)=1;
end

if x1>=-2-delta&&x1<=-1-delta
    ux1(1,1)=0.5*sin(pi*(x1-(-2-delta))/h1+0.5*pi)+0.5;
end

if x1>=-2-delta&&x1<=0-delta
    ux1(2,1)=0.5*sin(pi*(x1-(-1-delta))/h1+0.5*pi)+0.5;
end

if x1>=-1-delta&&x1<=1-delta
    ux1(3,1)=0.5*sin(pi*(x1-(0-delta))/h1+0.5*pi)+0.5;
end

if x1>=0-delta&&x1<=2-delta
    ux1(4,1)=0.5*sin(pi*(x1-(1-delta))/h1+0.5*pi)+0.5;
end

if x1>=1-delta&&x1<=2-delta
    ux1(5,1)=0.5*sin(pi*(x1-(2-delta))/h1+0.5*pi)+0.5;
end

if x1>2-delta
    ux1(5,1)=1;
end


h2=1;%%规则间距
if x2<=-2-delta
    ux2(1,1)=1;
end

if x2>=-2-delta&&x2<=-1-delta
    ux2(1,1)=0.5*sin(pi*(x2-(-2-delta))/h2+0.5*pi)+0.5;
end

if x2>=-2-delta&&x2<=0-delta
    ux2(2,1)=0.5*sin(pi*(x2-(-1-delta))/h2+0.5*pi)+0.5;
end

if x2>=-1-delta&&x2<=1-delta
    ux2(3,1)=0.5*sin(pi*(x2-(0-delta))/h2+0.5*pi)+0.5;
end

if x2>=0-delta&&x2<=2-delta
    ux2(4,1)=0.5*sin(pi*(x2-(1-delta))/h2+0.5*pi)+0.5;
end

if x2>=1-delta&&x2<=2-delta
    ux2(5,1)=0.5*sin(pi*(x2-(2-delta))/h2+0.5*pi)+0.5;
end

if x2>2-delta
    ux2(5,1)=1;
end

h3=1;%%规则间距
if x3<=-2-delta
    ux3(1,1)=1;
end

if x3>=-2-delta&&x3<=-1-delta
    ux3(1,1)=0.5*sin(pi*(x3-(-2-delta))/h3+0.5*pi)+0.5;
end

if x3>=-2-delta&&x3<=0-delta
    ux3(2,1)=0.5*sin(pi*(x3-(-1-delta))/h3+0.5*pi)+0.5;
end

if x3>=-1-delta&&x3<=1-delta
    ux3(3,1)=0.5*sin(pi*(x3-(0-delta))/h3+0.5*pi)+0.5;
end

if x3>=0-delta&&x3<=2-delta
    ux3(4,1)=0.5*sin(pi*(x3-(1-delta))/h3+0.5*pi)+0.5;
end

if x3>=1-delta&&x3<=2-delta
    ux3(5,1)=0.5*sin(pi*(x3-(2-delta))/h3+0.5*pi)+0.5;
end

if x3>2-delta
    ux3(5,1)=1;
end


%中心平均解模糊
Basic=0;
for i1=1:5
    for i2=1:5
        for i3=1:5
            Basic=Basic+ux1(i1,1)*ux2(i2,1)*ux3(i3,1);  
        end
    end
end

beta=zeros(5,5,5);
for i1=1:5
    for i2=1:5
        for i3=1:5
            beta(i1,i2,i3)=ux1(i1,1)*ux2(i2,1)*ux3(i3,1)/Basic;
        end
    end
end

wdot=zeros(5,5,5);
for i1=1:5
    for i2=1:5
        for i3=1:5
            wdot(i1,i2,i3)=w*beta(i1,i2,i3)*z3*u1;
        end
    end
end

end

== matlab function section_6_2_second_group/FUZZYB/fuzzy_logic_system1 ==
  data: aF output; x1 input; x2 input; x3 input; w input
function aF    = fcn(x1,x2,x3,w)
%%x1 5条模糊规则
delta=0.01;
ux1=zeros(5,1);
ux2=zeros(5,1);
ux3=zeros(5,1);
%%x1 5条模糊规则

h1=1;%%规则间距
if x1<=-2-delta
    ux1(1,1)=1;
end

if x1>=-2-delta&&x1<=-1-delta
    ux1(1,1)=0.5*sin(pi*(x1-(-2-delta))/h1+0.5*pi)+0.5;
end

if x1>=-2-delta&&x1<=0-delta
    ux1(2,1)=0.5*sin(pi*(x1-(-1-delta))/h1+0.5*pi)+0.5;
end

if x1>=-1-delta&&x1<=1-delta
    ux1(3,1)=0.5*sin(pi*(x1-(0-delta))/h1+0.5*pi)+0.5;
end

if x1>=0-delta&&x1<=2-delta
    ux1(4,1)=0.5*sin(pi*(x1-(1-delta))/h1+0.5*pi)+0.5;
end

if x1>=1-delta&&x1<=2-delta
    ux1(5,1)=0.5*sin(pi*(x1-(2-delta))/h1+0.5*pi)+0.5;
end

if x1>2-delta
    ux1(5,1)=1;
end


h2=1;%%规则间距
if x2<=-2-delta
    ux2(1,1)=1;
end

if x2>=-2-delta&&x2<=-1-delta
    ux2(1,1)=0.5*sin(pi*(x2-(-2-delta))/h2+0.5*pi)+0.5;
end

if x2>=-2-delta&&x2<=0-delta
    ux2(2,1)=0.5*sin(pi*(x2-(-1-delta))/h2+0.5*pi)+0.5;
end

if x2>=-1-delta&&x2<=1-delta
    ux2(3,1)=0.5*sin(pi*(x2-(0-delta))/h2+0.5*pi)+0.5;
end

if x2>=0-delta&&x2<=2-delta
    ux2(4,1)=0.5*sin(pi*(x2-(1-delta))/h2+0.5*pi)+0.5;
end

if x2>=1-delta&&x2<=2-delta
    ux2(5,1)=0.5*sin(pi*(x2-(2-delta))/h2+0.5*pi)+0.5;
end

if x2>2-delta
    ux2(5,1)=1;
end

h3=1;%%规则间距
if x3<=-2-delta
    ux3(1,1)=1;
end

if x3>=-2-delta&&x3<=-1-delta
    ux3(1,1)=0.5*sin(pi*(x3-(-2-delta))/h3+0.5*pi)+0.5;
end

if x3>=-2-delta&&x3<=0-delta
    ux3(2,1)=0.5*sin(pi*(x3-(-1-delta))/h3+0.5*pi)+0.5;
end

if x3>=-1-delta&&x3<=1-delta
    ux3(3,1)=0.5*sin(pi*(x3-(0-delta))/h3+0.5*pi)+0.5;
end

if x3>=0-delta&&x3<=2-delta
    ux3(4,1)=0.5*sin(pi*(x3-(1-delta))/h3+0.5*pi)+0.5;
end

if x3>=1-delta&&x3<=2-delta
    ux3(5,1)=0.5*sin(pi*(x3-(2-delta))/h3+0.5*pi)+0.5;
end

if x3>2-delta
    ux3(5,1)=1;
end



%中心平均解模糊
Basic=0;
for i1=1:5
    for i2=1:5
        for i3=1:5
            Basic=Basic+ux1(i1,1)*ux2(i2,1)*ux3(i3,1);
        end
    end
end

beta=zeros(5,5,5);
for i1=1:5
    for i2=1:5
        for i3=1:5
            beta(i1,i2,i3)=ux1(i1,1)*ux2(i2,1)*ux3(i3,1)/Basic;
        end
    end
end


aF=0;
for i1=1:5
    for i2=1:5
        for i3=1:5
            aF=aF+w(i1,i2,i3)*beta(i1,i2,i3); 
        end
    end
end

end

== matlab function section_6_2_second_group/FUZZYB/fuzzy_logic_system2 ==
  data: aF output; x1 input; x2 input; x3 input; w input
function aF    = fcn(x1,x2,x3,w)
%%x1 5条模糊规则
delta=0.01;
ux1=zeros(5,1);
ux2=zeros(5,1);
ux3=zeros(5,1);
%%x1 5条模糊规则

h1=1;%%规则间距
if x1<=-2-delta
    ux1(1,1)=1;
end

if x1>=-2-delta&&x1<=-1-delta
    ux1(1,1)=0.5*sin(pi*(x1-(-2-delta))/h1+0.5*pi)+0.5;
end

if x1>=-2-delta&&x1<=0-delta
    ux1(2,1)=0.5*sin(pi*(x1-(-1-delta))/h1+0.5*pi)+0.5;
end

if x1>=-1-delta&&x1<=1-delta
    ux1(3,1)=0.5*sin(pi*(x1-(0-delta))/h1+0.5*pi)+0.5;
end

if x1>=0-delta&&x1<=2-delta
    ux1(4,1)=0.5*sin(pi*(x1-(1-delta))/h1+0.5*pi)+0.5;
end

if x1>=1-delta&&x1<=2-delta
    ux1(5,1)=0.5*sin(pi*(x1-(2-delta))/h1+0.5*pi)+0.5;
end

if x1>2-delta
    ux1(5,1)=1;
end


h2=1;%%规则间距
if x2<=-2-delta
    ux2(1,1)=1;
end

if x2>=-2-delta&&x2<=-1-delta
    ux2(1,1)=0.5*sin(pi*(x2-(-2-delta))/h2+0.5*pi)+0.5;
end

if x2>=-2-delta&&x2<=0-delta
    ux2(2,1)=0.5*sin(pi*(x2-(-1-delta))/h2+0.5*pi)+0.5;
end

if x2>=-1-delta&&x2<=1-delta
    ux2(3,1)=0.5*sin(pi*(x2-(0-delta))/h2+0.5*pi)+0.5;
end

if x2>=0-delta&&x2<=2-delta
    ux2(4,1)=0.5*sin(pi*(x2-(1-delta))/h2+0.5*pi)+0.5;
end

if x2>=1-delta&&x2<=2-delta
    ux2(5,1)=0.5*sin(pi*(x2-(2-delta))/h2+0.5*pi)+0.5;
end

if x2>2-delta
    ux2(5,1)=1;
end

h3=1;%%规则间距
if x3<=-2-delta
    ux3(1,1)=1;
end

if x3>=-2-delta&&x3<=-1-delta
    ux3(1,1)=0.5*sin(pi*(x3-(-2-delta))/h3+0.5*pi)+0.5;
end

if x3>=-2-delta&&x3<=0-delta
    ux3(2,1)=0.5*sin(pi*(x3-(-1-delta))/h3+0.5*pi)+0.5;
end

if x3>=-1-delta&&x3<=1-delta
    ux3(3,1)=0.5*sin(pi*(x3-(0-delta))/h3+0.5*pi)+0.5;
end

if x3>=0-delta&&x3<=2-delta
    ux3(4,1)=0.5*sin(pi*(x3-(1-delta))/h3+0.5*pi)+0.5;
end

if x3>=1-delta&&x3<=2-delta
    ux3(5,1)=0.5*sin(pi*(x3-(2-delta))/h3+0.5*pi)+0.5;
end

if x3>2-delta
    ux3(5,1)=1;
end



%中心平均解模糊
Basic=0;
for i1=1:5
    for i2=1:5
        for i3=1:5
            Basic=Basic+ux1(i1,1)*ux2(i2,1)*ux3(i3,1);
        end
    end
end

beta=zeros(5,5,5);
for i1=1:5
    for i2=1:5
        for i3=1:5
            beta(i1,i2,i3)=ux1(i1,1)*ux2(i2,1)*ux3(i3,1)/Basic;
        end
    end
end


aF=0;
for i1=1:5
    for i2=1:5
        for i3=1:5
            aF=aF+w(i1,i2,i3)*beta(i1,i2,i3); 
        end
    end
end

end

== matlab function section_6_2_second_group/FUZZYB/fuzzy_logic_system3 ==
  data: aF output; x1 input; x2 input; x3 input; w input
function aF    = fcn(x1,x2,x3,w)
%%x1 5条模糊规则
delta=0.01;
ux1=zeros(5,1);
ux2=zeros(5,1);
ux3=zeros(5,1);
%%x1 5条模糊规则

h1=1;%%规则间距
if x1<=-2-delta
    ux1(1,1)=1;
end

if x1>=-2-delta&&x1<=-1-delta
    ux1(1,1)=0.5*sin(pi*(x1-(-2-delta))/h1+0.5*pi)+0.5;
end

if x1>=-2-delta&&x1<=0-delta
    ux1(2,1)=0.5*sin(pi*(x1-(-1-delta))/h1+0.5*pi)+0.5;
end

if x1>=-1-delta&&x1<=1-delta
    ux1(3,1)=0.5*sin(pi*(x1-(0-delta))/h1+0.5*pi)+0.5;
end

if x1>=0-delta&&x1<=2-delta
    ux1(4,1)=0.5*sin(pi*(x1-(1-delta))/h1+0.5*pi)+0.5;
end

if x1>=1-delta&&x1<=2-delta
    ux1(5,1)=0.5*sin(pi*(x1-(2-delta))/h1+0.5*pi)+0.5;
end

if x1>2-delta
    ux1(5,1)=1;
end


h2=1;%%规则间距
if x2<=-2-delta
    ux2(1,1)=1;
end

if x2>=-2-delta&&x2<=-1-delta
    ux2(1,1)=0.5*sin(pi*(x2-(-2-delta))/h2+0.5*pi)+0.5;
end

if x2>=-2-delta&&x2<=0-delta
    ux2(2,1)=0.5*sin(pi*(x2-(-1-delta))/h2+0.5*pi)+0.5;
end

if x2>=-1-delta&&x2<=1-delta
    ux2(3,1)=0.5*sin(pi*(x2-(0-delta))/h2+0.5*pi)+0.5;
end

if x2>=0-delta&&x2<=2-delta
    ux2(4,1)=0.5*sin(pi*(x2-(1-delta))/h2+0.5*pi)+0.5;
end

if x2>=1-delta&&x2<=2-delta
    ux2(5,1)=0.5*sin(pi*(x2-(2-delta))/h2+0.5*pi)+0.5;
end

if x2>2-delta
    ux2(5,1)=1;
end

h3=1;%%规则间距
if x3<=-2-delta
    ux3(1,1)=1;
end

if x3>=-2-delta&&x3<=-1-delta
    ux3(1,1)=0.5*sin(pi*(x3-(-2-delta))/h3+0.5*pi)+0.5;
end

if x3>=-2-delta&&x3<=0-delta
    ux3(2,1)=0.5*sin(pi*(x3-(-1-delta))/h3+0.5*pi)+0.5;
end

if x3>=-1-delta&&x3<=1-delta
    ux3(3,1)=0.5*sin(pi*(x3-(0-delta))/h3+0.5*pi)+0.5;
end

if x3>=0-delta&&x3<=2-delta
    ux3(4,1)=0.5*sin(pi*(x3-(1-delta))/h3+0.5*pi)+0.5;
end

if x3>=1-delta&&x3<=2-delta
    ux3(5,1)=0.5*sin(pi*(x3-(2-delta))/h3+0.5*pi)+0.5;
end

if x3>2-delta
    ux3(5,1)=1;
end



%中心平均解模糊
Basic=0;
for i1=1:5
    for i2=1:5
        for i3=1:5
            Basic=Basic+ux1(i1,1)*ux2(i2,1)*ux3(i3,1);
        end
    end
end

beta=zeros(5,5,5);
for i1=1:5
    for i2=1:5
        for i3=1:5
            beta(i1,i2,i3)=ux1(i1,1)*ux2(i2,1)*ux3(i3,1)/Basic;
        end
    end
end


aF=0;
for i1=1:5
    for i2=1:5
        for i3=1:5
            aF=aF+w(i1,i2,i3)*beta(i1,i2,i3); 
        end
    end
end

end

== matlab function section_6_2_second_group/controller ==
  data: aF1 input; aF2 input; aF3 input; xdt input; xd input; u1 output; u2 output; u3 output; x11 input; x12 input; x13 input; x21 input; x22 input; x23 input; x31 input; x32 input; x33 input; Kv11 input; Kv12 input; z11 output; z12 output; z13 output; z21 output; z22 output; z23 output; z31 output; z32 output; z33 output; Kv21 input; Kv22 input; Kv31 input; Kv32 input; delta1 input; delta2 input; delta3 input; dag input; BF1 input; BF2 input; BF3 input
function [u1,u2,u3,z11,z12,z13,z21,z22,z23,z31,z32,z33]  = fcn(aF1,aF2,aF3,xdt,xd,x11,x12,x13,x21,x22,x23,x31,x32,x33,Kv11,Kv12,Kv21,Kv22,Kv31,Kv32,delta1,delta2,delta3,dag,BF1,BF2,BF3)
wa11=0;
wa12=0;
wa13=0;
wb1=4;
wa21=6;
wa22=0;
wa23=0;
wb2=0;
wa31=0;
wa32=5;
wa33=0;
wb3=0;
AF1=zeros(3,3);
for i=1:3
    for j=1:3
        AF1(i,j)=aF1(i+3*(j-1));
%         AF1(i,j)=1;
    end
end
AF2=zeros(3,3);
for i=1:3
    for j=1:3
        AF2(i,j)=aF2(i+3*(j-1));
%         AF2(i,j)=1;
    end
end
AF3=zeros(3,3);
for i=1:3
    for j=1:3
        AF3(i,j)=aF3(i+3*(j-1));
%         AF3(i,j)=1;
    end
end
% AF1(1,1)=0;
% AF1(1,3)=0;
AF1(1,2)=6;
AF1(2,3)=6;
% BF1=1;
AF2(1,2)=6;
AF2(2,3)=6;
% BF2=1;
AF3(1,2)=6;
AF3(2,3)=6;
% BF3=1;

% delta11=(abs(AF1(1,1))+abs(AF1(1,2))+abs(AF1(1,3)))*1;
% delta12=(abs(AF1(2,1))+abs(AF1(2,2))+abs(AF1(2,3)))*1;
% delta13=(abs(AF1(3,1))+abs(AF1(3,2))+abs(AF1(3,3)))*1;
% delta21=(abs(AF2(1,1))+abs(AF2(1,2))+abs(AF2(1,3)))*1;
% delta22=(abs(AF2(2,1))+abs(AF2(2,2))+abs(AF2(2,3)))*1;
% delta23=(abs(AF2(3,1))+abs(AF2(3,2))+abs(AF2(3,3)))*1;
% delta31=(abs(AF3(1,1))+abs(AF3(1,2))+abs(AF3(1,3)))*1;
% delta32=(abs(AF3(2,1))+abs(AF3(2,2))+abs(AF3(2,3)))*1;
% delta33=(abs(AF3(3,1))+abs(AF3(3,2))+abs(AF3(3,3)))*1;


z11=wa11*(x11-x11)+wa12*(x11-x21)+wa13*(x11-x31)+wb1*(x11-xd);
% K1=z11/dag^2*delta1+z11/dag^2*(delta11^2/2+1/(wb1+wa11+wa12+wa13)*(delta12^2/2+delta13^2/2))+z11/dag^2*1/(wb1+wa11+wa12+wa13)*(wa11*delta11^2/2+wa12*delta21^2/2+wa13*delta31^2/2);
K1=z11/dag^2*delta1;
% K1=0;
v11=-1/AF1(1,2)*((z11/2+K1+AF1(1,1)*x11+AF1(1,3)*x13)-1/(wb1+wa11+wa12+wa13)*(wa11*(AF1(1,1)*x11+AF1(1,2)*x12+AF1(1,3)*x13)+wa12*(AF2(1,1)*x21+AF2(1,2)*x22+AF2(1,3)*x23)+wa13*(AF3(1,1)*x31+AF3(1,2)*x32+AF3(1,3)*x33)+(wa11+wa12+wa13)*z11/2)-wb1/(wb1+wa11+wa12+wa13)*xdt);
z12=x12-v11;
% sat12=0;
% if z12<0.1
%     sat12=z12/0.1;
% else
%     sat12=sign(z12);
% end
% sat12=sign(z12);
v12=-1/AF1(2,3)*(AF1(2,1)*x11+AF1(2,2)*x12+z12/2+(wb1+wa11+wa12+wa13)*AF1(1,2)*z11+Kv11*z12);
% v12=-1/AF1(2,3)*(AF1(2,1)*x11+AF1(2,2)*x12+z12/2+(wb1+wa11+wa12+wa13)*AF1(1,2)*z11+Kv11*sat12);
z13=x13-v12;
% sat13=0;
% if z13<0.1
%     sat13=z13/0.1;
% else
%     sat13=sign(z13);
% end
% sat13=sign(z13);
u1=-1/BF1*(AF1(3,1)*x11+AF1(3,2)*x12+AF1(3,3)*x13+z13/2+AF1(2,3)*z12+Kv12*z13);
% u1=-1/BF1*(AF1(3,1)*x11+AF1(3,2)*x12+AF1(3,3)*x13+z13/2+AF1(2,3)*z12+Kv12*sat13);
u1=20*tanh(u1/20);


z21=wa21*(x21-x11)+wa22*(x21-x21)+wa23*(x21-x31)+wb2*(x21-xd);
% K2=z21/dag^2*delta2+z21/dag^2*(delta21^2/2+1/(wb2+wa21+wa22+wa23)*(delta22^2/2+delta23^2/2))+z21/dag^2*1/(wb2+wa21+wa22+wa23)*(wa21*delta11^2/2+wa22*delta21^2/2+wa23*delta31^2/2);
K2=z21/dag^2*delta2;
% K2=0;
v21=-1/AF2(1,2)*((z21/2+K2+AF2(1,1)*x21+AF2(1,3)*x23)-1/(wb2+wa21+wa22+wa23)*(wa21*(AF1(1,1)*x11+AF1(1,2)*x12+AF1(1,3)*x13)+wa22*(AF2(1,1)*x21+AF2(1,2)*x22+AF2(1,3)*x23)+wa23*(AF3(1,1)*x31+AF3(1,2)*x32+AF3(1,3)*x33)+(wa21+wa22+wa23)*z21/2)-wb2/(wb2+wa21+wa22+wa23)*xdt);
z22=x22-v21;
% sat22=0;
% if z22<0.1
%     sat22=z22/0.1;
% else
%     sat22=sign(z22);
% end
% sat22=sign(z22);
v22=-1/AF2(2,3)*(AF2(2,1)*x21+AF2(2,2)*x22+z22/2+(wb2+wa21+wa22+wa23)*AF2(1,2)*z21+Kv21*z22);
% v22=-1/AF2(2,3)*(AF2(2,1)*x21+AF2(2,2)*x22+z22/2+(wb2+wa21+wa22+wa23)*AF2(1,2)*z21+Kv21*sat22);
z23=x23-v22;
% sat23=0;
% if z23<0.1
%     sat23=z23/0.1;
% else
%     sat23=sign(z23);
% end
% sat23=sign(z23);
u2=-1/BF2*(AF2(3,1)*x21+AF2(3,2)*x22+AF2(3,3)*x23+z23/2+AF2(2,3)*z22+Kv22*z23);
% u2=-1/BF2*(AF2(3,1)*x21+AF2(3,2)*x22+AF2(3,3)*x23+z23/2+AF2(2,3)*z22+Kv22*sat23);
u2=20*tanh(u2/20);

z31=wa31*(x31-x11)+wa32*(x31-x21)+wa33*(x31-x31)+wb3*(x31-xd);
% K3=z31/dag^2*delta3+z31/dag^2*(delta31^2/2+1/(wb3+wa31+wa32+wa33)*(delta32^2/2+delta33^2/2))+z31/dag^2*1/(wb3+wa31+wa32+wa33)*(wa31*delta11^2/2+wa32*delta21^2/2+wa33*delta31^2/2);
K3=z31/dag^2*delta3;
% K3=0;
v31=-1/AF3(1,2)*((z31/2+K3+AF3(1,1)*x31+AF3(1,3)*x33)-1/(wb3+wa31+wa32+wa33)*(wa31*(AF1(1,1)*x11+AF1(1,2)*x12+AF1(1,3)*x13)+wa32*(AF2(1,1)*x21+AF2(1,2)*x22+AF2(1,3)*x23)+wa33*(AF3(1,1)*x31+AF3(1,2)*x32+AF3(1,3)*x33)+(wa31+wa32+wa33)*z31/2)-wb3/(wb3+wa31+wa32+wa33)*xdt);
z32=x32-v31;
% sat32=0;
% if z32<0.1
%     sat32=z32/0.1;
% else
%     sat32=sign(z32);
% end
% sat32=sign(z32);
v32=-1/AF3(2,3)*(AF3(2,1)*x31+AF3(2,2)*x32+z32/2+(wb3+wa31+wa32+wa33)*AF3(1,2)*z31+Kv31*z32);
% v32=-1/AF3(2,3)*(AF3(2,1)*x31+AF3(2,2)*x32+z32/2+(wb3+wa31+wa32+wa33)*AF3(1,2)*z31+Kv31*sat32);
z33=x33-v32;
% sat33=0;
% if z33<0.1
%     sat33=z33/0.1;
% else
%     sat33=sign(z33);
% end
% sat33=sign(z33);
u3=-1/BF3*(AF3(3,1)*x31+AF3(3,2)*x32+AF3(3,3)*x33+z33/2+AF3(2,3)*z32+Kv32*z33);
% u3=-1/BF3*(AF3(3,1)*x31+AF3(3,2)*x32+AF3(3,3)*x33+z33/2+AF3(2,3)*z32+Kv32*sat33);
u3=20*tanh(u3/20);


end

== matlab function section_6_2_second_group/Kv11_adaptive ==
  data: w input; z12 input; Kv_dot output
function Kv_dot  = fcn(w,z12)
Kv_dot=w*abs(z12);
end

== matlab function section_6_2_second_group/Leader ==
  data: x input; xdot output; t input
function xdot  = fcn(x,t)

xdot=-1.2*x+0.5*cos(0.5*t+3)+3*(t^2)*exp(-t)-0.5;
% xdot=0.5*cos(0.5*t);
end

== matlab function section_6_2_second_group/follower2 ==
  data: x1 input; x2 input; x3 input; x1dot output; u2 input; x2dot output; x3dot output
function [x1dot,x2dot,x3dot] = fcn(x1,x2,x3,u2)

f11=-x1+2*tanh(x3+10*x2^2);
f12=x3+6*tanh(20*x3^2);
f13=exp(x1*x2)+9; 

g11=0.5*sin(x1+x3);
g12=x2*sin(0.2/(3+x1^2+x3^2));
g13=x3^2/(1+x1^2+x2^2)+0.1*exp(-u2^2);

x1dot=f11*sin(x2)+g11;
x2dot=f12*x3+g12;
x3dot=f13*u2+g13;


% x1dot=x1+x2+x3;
% x2dot=x1+x2+x3;
% x3dot=x1+x2+x3+u2;
      
end

== matlab function section_6_2_second_group/FUZZY1/3D-2D2 ==
  data: y output; x input
function y  = fcn(x)
y=zeros(25,5);

for i=1:5
    for j=1:5
        for k=1:5
            y(5*(k-1)+i,j)=x(i,j,k);
        end
    end
end


end

== matlab function section_6_2_second_group/follower3 ==
  data: x1 input; x2 input; x3 input; x1dot output; u3 input; x2dot output; x3dot output
function [x1dot,x2dot,x3dot] = fcn(x1,x2,x3,u3)

% f11=x1+2*tanh(x3+10*x2^2);
% f12=cos(x3)+6*tanh(x1+10*x3^2);
% f13=exp(x1*x2)+170*tanh(x2+10*u3^2); 
% 
% g11=x3^2/(1+x1^2+x2^2);
% g12=x2*sin(0.2/(3+x1^2+x3^2));
% g13=x3^2/(1+x1^2+x2^2)+0.1*sin(u3);
% 
% x1dot=f11*sin(x2)+g11+sin(x1+x2+x3);
% x2dot=f12*x3+g12+sin(x1+x2+x3);
% x3dot=f13*sin(u3/15)+g13+sin(x1+x2+x3);

x1dot=sin(x1+x2+x3)+2*x2+x3;
x2dot=sin(x1+x2+x3)+x2+2*x3;
x3dot=sin(x1+x2+x3)+3*u3;
      
end

== matlab function section_6_2_second_group/FUZZY1/2D-3D1 ==
  data: y output; x input
function y  = fcn(x)
y=zeros(5,5,5);

for i=1:5
    for j=1:5
        for k=1:5
            y(i,j,k)=x(5*(k-1)+i,j);
        end
    end
end

end

== matlab function section_6_2_second_group/FUZZY1/fuzzy_adaptive_law2 ==
  data: wdot output; x1 input; x2 input; x3 input; zz input; w input
function wdot   = fcn(x1,x2,x3,zz,w)
delta=0.01;
ux1=zeros(5,1);
ux2=zeros(5,1);
ux3=zeros(5,1);
%%x1 5条模糊规则

z=zeros(5,6);
for j=1:5
    z(j,1)=-2+j-delta;
end
for j=6:10
    z(j-5,2)=-2+(j-5)-delta;
end
for j=11:15
    z(j-10,3)=-2+(j-10)-delta;
end

h1=1;%%规则间距
if x1<=-2-delta
    ux1(1,1)=1;
end

if x1>=-2-delta&&x1<=-1-delta
    ux1(1,1)=0.5*sin(pi*(x1-(-2-delta))/h1+0.5*pi)+0.5;
end

if x1>=-2-delta&&x1<=0-delta
    ux1(2,1)=0.5*sin(pi*(x1-(-1-delta))/h1+0.5*pi)+0.5;
end

if x1>=-1-delta&&x1<=1-delta
    ux1(3,1)=0.5*sin(pi*(x1-(0-delta))/h1+0.5*pi)+0.5;
end

if x1>=0-delta&&x1<=2-delta
    ux1(4,1)=0.5*sin(pi*(x1-(1-delta))/h1+0.5*pi)+0.5;
end

if x1>=1-delta&&x1<=2-delta
    ux1(5,1)=0.5*sin(pi*(x1-(2-delta))/h1+0.5*pi)+0.5;
end

if x1>2-delta
    ux1(5,1)=1;
end


h2=1;%%规则间距
if x2<=-2-delta
    ux2(1,1)=1;
end

if x2>=-2-delta&&x2<=-1-delta
    ux2(1,1)=0.5*sin(pi*(x2-(-2-delta))/h2+0.5*pi)+0.5;
end

if x2>=-2-delta&&x2<=0-delta
    ux2(2,1)=0.5*sin(pi*(x2-(-1-delta))/h2+0.5*pi)+0.5;
end

if x2>=-1-delta&&x2<=1-delta
    ux2(3,1)=0.5*sin(pi*(x2-(0-delta))/h2+0.5*pi)+0.5;
end

if x2>=0-delta&&x2<=2-delta
    ux2(4,1)=0.5*sin(pi*(x2-(1-delta))/h2+0.5*pi)+0.5;
end

if x2>=1-delta&&x2<=2-delta
    ux2(5,1)=0.5*sin(pi*(x2-(2-delta))/h2+0.5*pi)+0.5;
end

if x2>2-delta
    ux2(5,1)=1;
end

h3=1;%%规则间距
if x3<=-2-delta
    ux3(1,1)=1;
end

if x3>=-2-delta&&x3<=-1-delta
    ux3(1,1)=0.5*sin(pi*(x3-(-2-delta))/h3+0.5*pi)+0.5;
end

if x3>=-2-delta&&x3<=0-delta
    ux3(2,1)=0.5*sin(pi*(x3-(-1-delta))/h3+0.5*pi)+0.5;
end

if x3>=-1-delta&&x3<=1-delta
    ux3(3,1)=0.5*sin(pi*(x3-(0-delta))/h3+0.5*pi)+0.5;
end

if x3>=0-delta&&x3<=2-delta
    ux3(4,1)=0.5*sin(pi*(x3-(1-delta))/h3+0.5*pi)+0.5;
end

if x3>=1-delta&&x3<=2-delta
    ux3(5,1)=0.5*sin(pi*(x3-(2-delta))/h3+0.5*pi)+0.5;
end

if x3>2-delta
    ux3(5,1)=1;
end


%中心平均解模糊
Basic=0;
for i1=1:5
    for i2=1:5
        for i3=1:5
            Basic=Basic+ux1(i1,1)*ux2(i2,1)*ux3(i3,1);  
        end
    end
end

beta=zeros(5,5,5);
for i1=1:5
    for i2=1:5
        for i3=1:5
            beta(i1,i2,i3)=ux1(i1,1)*ux2(i2,1)*ux3(i3,1)/Basic;
        end
    end
end

wdot=zeros(5,5,5);
for i1=1:5
    for i2=1:5
        for i3=1:5
            wdot(i1,i2,i3)=w*beta(i1,i2,i3)*zz*z(i3,1);
        end
    end
end

end

== matlab function section_6_2_second_group/FUZZY1/3D-2D1 ==
  data: y output; x input
function y  = fcn(x)
y=zeros(25,5);

for i=1:5
    for j=1:5
        for k=1:5
            y(5*(k-1)+i,j)=x(i,j,k);
        end
    end
end


end
